simulink model "hybrid_new_eq_circuit_pascal5_single_shot_stack"  (R2019a)
settings: Solver=FixedStepAuto  StartTime=0.0  StopTime=sim_time  FixedStep=resolution  MinStep=0.001  RelTol=1e-4  EnableMultiTasking=on
values from neighbouring files (symbols this model uses):
  amps_in = double(amps_in)    [Sc.m]    (also in sc_model_single_shot_stack.m; test.m = 0; workspace_nedc_basic_sc.mat = 0; workspace_test_model.mat = 0)
  batt_c = [0.25 0.25 0.25 0.25 0.25 0.25 0.25]    [workspace_test_model.mat]
  batt_r = [1 1 1 1 1 1 1 1]    [workspace_test_model.mat]
  resolution = double(resolution)    [Sc.m]    (also in sc_model_single_shot.m = 0.1; sc_model_single_shot_stack.m = 0.1; workspace_test_model.mat = 10)
  tStep = resolution    (= 0.1)    [Sc.m]    (also in testHyb.m = 10; workspace_test_model.mat = 10)
undefined symbols (not defined in the file or in its folder): cCap, cR
libraries: powerlib x525, simulink x9
(part 1 of 8)
settings Model: Creator=ttsh  LastModifiedBy=ttsh
settings SolverCC: ZeroCrossAlgorithm=Adaptive  AlgebraicLoopSolver=LineSearch  SolverResetMethod=Robust
settings DataIOCC: LimitDataPoints=on  SaveFormat=Array  ReturnWorkspaceOutputs=off
settings OptimizationCC: LifeSpan=inf
settings DebuggingCC: SolverPrmCheckMsg=warning  UnconnectedInputMsg=none  UnconnectedOutputMsg=none  UnconnectedLineMsg=none  AllowSymbolicDim=off  SFUnexpectedBacktrackingDiag=warning  SFNoUnconditionalDefaultTransitionDiag=warning  SFExecutionAtInitializationDiag=none  ArithmeticOperatorsInVariantConditions=warning
settings HardwareCC: ProdBitPerPointer=32  ProdBitPerSizeT=32  ProdBitPerPtrDiffT=32  ProdLargestAtomicFloat=None  ProdIntDivRoundTo=Undefined  ProdEndianess=Unspecified  ProdWordSize=32  ProdHWDeviceType=32-bit Generic
settings ModelReferenceCC: PropagateSignalLabelsOutOfModel=off
settings SFSimCC: SimUseLocalCustomCode=off
settings RTWCC: RTWUseLocalCustomCode=off
settings CodeAppCC: StateflowObjectComments=on
settings GRTTargetCC: TargetLangStandard=C89/C90 (ANSI)  GeneratePreprocessorConditionals=Disable all
settings ConfigComp: CovMetricSettings=dw  CovHtmlReporting=on  CovSaveCumulativeToWorkspaceVar=on  CovSaveSingleToWorkspaceVar=on  CovExternalEMLEnable=off  CovSFcnEnable=off
settings SimscapeCC: SimscapeNormalizeSystem=off

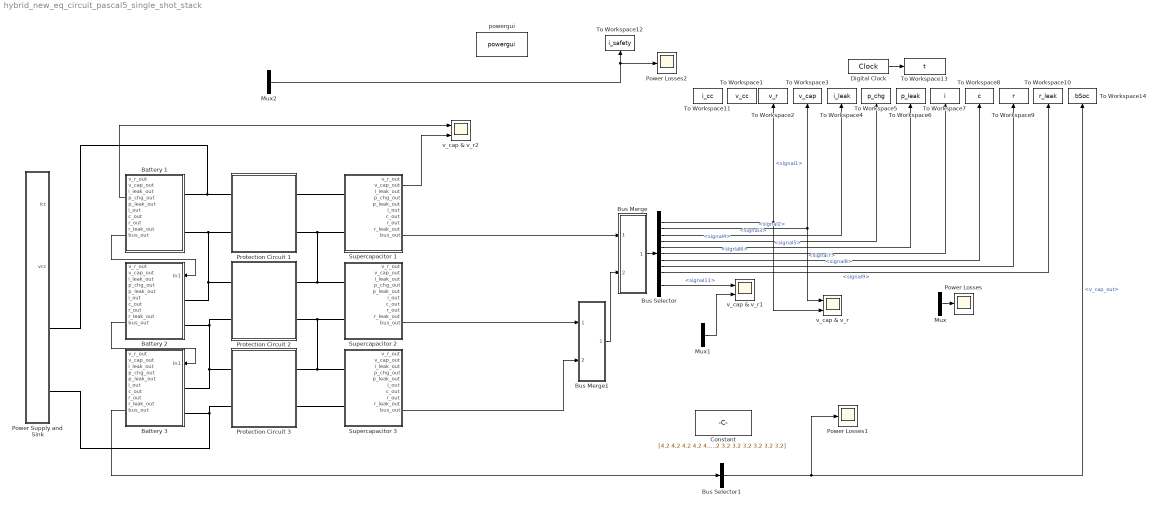
== system hybrid_new_eq_circuit_pascal5_single_shot_stack ==
  Battery 1 : Subsystem  mask{r=batt_r, c=batt_c, v_init=bv_init(end, :, 1), r_leak=inf}
      mask prompts: r "R /ohm (inf for disabled)"; c "Capacitance /F"; v_init "Initial capacitor voltage"; r_leak "R Leak (inf for disabled)"
  Battery 2 : Subsystem  mask{r=batt_r, c=batt_c, v_init=bv_init(end, :, 2), r_leak=inf}
      mask prompts: r "R /ohm (inf for disabled)"; c "Capacitance /F"; v_init "Initial capacitor voltage"; r_leak "R Leak (inf for disabled)"
  Battery 3 : Subsystem  mask{r=batt_r, c=batt_c, v_init=bv_init(end, :, 3), r_leak=inf}
      mask prompts: r "R /ohm (inf for disabled)"; c "Capacitance /F"; v_init "Initial capacitor voltage"; r_leak "R Leak (inf for disabled)"
  Bus Selector : BusSelector  OutputSignals=signal1,signal2,signal3,signal4,signal5,signal6,signal7,signal8,signal9,signal10,signal11
  Bus Selector1 : BusSelector  OutputSignals=v_cap_out
  Bus Merge : Subsystem
  Bus Merge1 : Subsystem
  Constant : Constant  Value=[4.2 4.2 4.2 4.2 4.2 4.2 4.2 4.2 4.2 4.2 4.2 4.2 4.2 4.2 3.2 3.2 3.2 3.2 3.2 3.2 3.2]
  Digital Clock : DigitalClock  SampleTime=resolution
  Mux : Mux  Inputs=2
  Mux1 : Mux  Inputs=2
  Mux2 : Mux  Inputs=3
  Power Losses : Scope
  Power Losses1 : Scope
  Power Losses2 : Scope
  Power Supply and Sink : Subsystem  mask{v_ovp=24}
      mask prompts: v_ovp "V OVP"
  Protection Circuit 1 : Subsystem  mask{r=10, d=0.01, v_cut=8.1, v_min=0, k=off}
      mask prompts: r "Series resistance"; d "Rate limit"; v_cut "v cutoff"; v_min "v min"; k "Enable"
  Protection Circuit 2 : Subsystem  mask{r=10, d=0.01, v_cut=8.1, v_min=0, k=off}
      mask prompts: r "Series resistance"; d "Rate limit"; v_cut "v cutoff"; v_min "v min"; k "Enable"
  Protection Circuit 3 : Subsystem  mask{r=10, d=0.01, v_cut=8.1, v_min=0, k=off}
      mask prompts: r "Series resistance"; d "Rate limit"; v_cut "v cutoff"; v_min "v min"; k "Enable"
  Supercapacitor 1 : Subsystem  mask{r_leak=inf, c=cCap, r=cR, ord=5, v_init1=v_init(end, 1, 1), v_init2=v_init(end, 2, 1), v_init3=v_init(end, 3, 1), v_init4=v_init(end, 4, 1), v_init5=v_init(end, 5, 1)}
      mask prompts: r_leak "R Leak /ohm (inf for disabled)"; c "Capacitance /F"; r "Resistance"; ord "Elements (pascal order)"; v_init1 "Initial capacitor voltage"; v_init2 "Initial capacitor voltage"; v_init3 "Initial capacitor voltage"; v_init4 "Initial capacitor voltage"; v_init5 "Initial capacitor voltage"
  Supercapacitor 2 : Subsystem  mask{r_leak=inf, c=cCap, r=cR, ord=5, v_init1=v_init(end, 1, 2), v_init2=v_init(end, 2, 2), v_init3=v_init(end, 3, 2), v_init4=v_init(end, 4, 2), v_init5=v_init(end, 5, 2)}
      mask prompts: r_leak "R Leak /ohm (inf for disabled)"; c "Capacitance /F"; r "Resistance"; ord "Elements (pascal order)"; v_init1 "Initial capacitor voltage"; v_init2 "Initial capacitor voltage"; v_init3 "Initial capacitor voltage"; v_init4 "Initial capacitor voltage"; v_init5 "Initial capacitor voltage"
  Supercapacitor 3 : Subsystem  mask{r_leak=inf, c=cCap, r=cR, ord=5, v_init1=v_init(end, 1, 3), v_init2=v_init(end, 2, 3), v_init3=v_init(end, 3, 3), v_init4=v_init(end, 4, 3), v_init5=v_init(end, 5, 3)}
      mask prompts: r_leak "R Leak /ohm (inf for disabled)"; c "Capacitance /F"; r "Resistance"; ord "Elements (pascal order)"; v_init1 "Initial capacitor voltage"; v_init2 "Initial capacitor voltage"; v_init3 "Initial capacitor voltage"; v_init4 "Initial capacitor voltage"; v_init5 "Initial capacitor voltage"
  To Workspace1 : ToWorkspace  VariableName=v_cc  SampleTime=-1
      settings: Save2DSignal=2-D array (concatenate along first dimension)
  To Workspace10 : ToWorkspace  VariableName=r_leak  SampleTime=-1
  To Workspace11 : ToWorkspace  VariableName=i_cc  SampleTime=-1
      settings: Save2DSignal=2-D array (concatenate along first dimension)
  To Workspace12 : ToWorkspace  VariableName=i_safety  SampleTime=-1
      settings: Save2DSignal=2-D array (concatenate along first dimension)
  To Workspace13 : ToWorkspace  VariableName=t  SampleTime=-1
      settings: Save2DSignal=2-D array (concatenate along first dimension)
  To Workspace14 : ToWorkspace  VariableName=bSoc  SampleTime=-1
  To Workspace2 : ToWorkspace  VariableName=v_r  SampleTime=-1
  To Workspace3 : ToWorkspace  VariableName=v_cap  SampleTime=-1
  To Workspace4 : ToWorkspace  VariableName=i_leak  SampleTime=-1
  To Workspace5 : ToWorkspace  VariableName=p_chg  SampleTime=-1
  To Workspace6 : ToWorkspace  VariableName=p_leak  SampleTime=-1
  To Workspace7 : ToWorkspace  VariableName=i  SampleTime=-1
  To Workspace8 : ToWorkspace  VariableName=c  SampleTime=-1
  To Workspace9 : ToWorkspace  VariableName=r  SampleTime=-1
  powergui : powerlib/powergui  Priority=1  SimulationMode=Discrete  SampleTime=tStep  frequency=60  Iterations=50  frequencyindice=0  Pbase=100e6  ErrMax=1e-4  UnitsV=V  UnitsW=W  buscounter=0  FunctionMessages=on  echomessages=off  EnableUseOfTLC=off  CurrentSourceSwitches=on  DisableSnubberDevices=on  DisableRonSwitches=on  DisableVfSwitches=on  DisplayEquations=off  AutomaticDiscreteSolvers=off  SolverType=Tustin  Interpol=off  ExternalGateDelay=off  methode=off  Ts=0  x0status=blocks  SPID=off  SwTol=0  HookPort=off  NonlinearTolerance=0  nMaxIteration=15  ContinueOnMaxIteration=off  RestoreLinks=warning  ResistiveCurrentMeasurement=off  Frange=[0:2:500]  Ylog=off  Xlog=on  ShowGrid=off  save=off  variable=ZData  structure=0  ZoomFFT=off  StartTime=0.0  cycles=1  DisplayStyle=1  fundamental=60  FreqAxis=off  MaxFrequency=1000  frequencyindicesteady=1  RmsSteady=1  display=off
      settings: SourceProductName=Simscape Electrical
  v_cap & v_r : Scope  NumInputPorts=2
  v_cap & v_r1 : Scope  NumInputPorts=2
  v_cap & v_r2 : Scope  NumInputPorts=2
  wires:
  Mux/1 -> Power Losses/1
  Supercapacitor 1/10(bus_out) -> Bus Merge/1(bus_1_in)
  Bus Merge/1(bus_out) -> Bus Selector/1
  Bus Selector/1 -> v_cap & v_r/2, To Workspace2/1  "<signal1>"
  Bus Selector/2 -> v_cap & v_r/1, To Workspace3/1  "<signal2>"
  Bus Selector/3 -> To Workspace4/1  "<signal3>"
  Bus Selector/4 -> To Workspace5/1  "<signal4>"
  Bus Selector/5 -> To Workspace6/1  "<signal5>"
  Bus Selector/6 -> To Workspace7/1  "<signal6>"
  Bus Selector/7 -> To Workspace8/1  "<signal7>"
  Bus Selector/8 -> To Workspace9/1  "<signal8>"
  Bus Selector/9 -> To Workspace10/1  "<signal9>"
  Bus Selector/11 -> v_cap & v_r1/1  "<signal11>"
  Supercapacitor 2/10(bus_out) -> Bus Merge1/1(bus_1_in)
  Supercapacitor 3/10(bus_out) -> Bus Merge1/2(bus_2_in)
  Bus Merge1/1(bus_out) -> Bus Merge/2(bus_2_in)
  Mux1/1 -> v_cap & v_r1/2
  Mux2/1 -> Power Losses2/1, To Workspace12/1
  Digital Clock/1 -> To Workspace13/1
  Supercapacitor 1/2(v_cap_out) -> v_cap & v_r2/2
  Battery 1/4(p_chg_out) -> v_cap & v_r2/1
  Battery 1/10(bus_out) -> Battery 2/1(In1)
  Battery 2/10(bus_out) -> Battery 3/1(In1)
  Battery 3/10(bus_out) -> Bus Selector1/1
  Bus Selector1/1 -> To Workspace14/1, Power Losses1/1  "<v_cap_out>"
  connections:
  Power Supply and Sink/RConn1 -- Battery 1/LConn1 -- Protection Circuit 1/LConn1
  Protection Circuit 2/LConn1 -- Battery 1/LConn2 -- Protection Circuit 1/LConn2 -- Battery 2/LConn1
  Protection Circuit 1/RConn1 -- Supercapacitor 1/LConn1
  Protection Circuit 2/RConn1 -- Supercapacitor 2/LConn1 -- Supercapacitor 1/LConn2 -- Protection Circuit 1/RConn2
  Protection Circuit 2/LConn2 -- Battery 2/LConn2 -- Battery 3/LConn1 -- Protection Circuit 3/LConn1
  Power Supply and Sink/RConn2 -- Battery 3/LConn2 -- Protection Circuit 3/LConn2
  Protection Circuit 2/RConn2 -- Supercapacitor 2/LConn2 -- Supercapacitor 3/LConn1 -- Protection Circuit 3/RConn1
  Supercapacitor 3/LConn2 -- Protection Circuit 3/RConn2

== system hybrid_new_eq_circuit_pascal5_single_shot_stack/Battery 1 ==
  note: 1x 550R
  Bus Creator : BusCreator  Inputs=11
  Constant : Constant
  Series RLC Branch1 : powerlib/Elements/Series RLC Branch  LConnTagsString=__new0  RConnTagsString=__new0  BranchType=R  Resistance=r(8)  Inductance=1e-3  SetiL0=off  InitialCurrent=0  Capacitance=1e-6  Setx0=off  InitialVoltage=0  Measurements=None
      settings: SourceProductName=Simscape Electrical
  Series RLC Branch2 : powerlib/Elements/Series RLC Branch  LConnTagsString=__new0  RConnTagsString=__new0  BranchType=R  Resistance=r(1)  Inductance=1e-3  SetiL0=off  InitialCurrent=0  Capacitance=1e-6  Setx0=off  InitialVoltage=0  Measurements=None
      settings: SourceProductName=Simscape Electrical
  Series RLC Branch3 : powerlib/Elements/Series RLC Branch  LConnTagsString=__new0  RConnTagsString=__new0  BranchType=R  Resistance=r(2)  Inductance=1e-3  SetiL0=off  InitialCurrent=0  Capacitance=1e-6  Setx0=off  InitialVoltage=0  Measurements=None
      settings: SourceProductName=Simscape Electrical
  Series RLC Branch4 : powerlib/Elements/Series RLC Branch  LConnTagsString=__new0  RConnTagsString=__new0  BranchType=R  Resistance=r(3)  Inductance=1e-3  SetiL0=off  InitialCurrent=0  Capacitance=1e-6  Setx0=off  InitialVoltage=0  Measurements=None
      settings: SourceProductName=Simscape Electrical
  Subsystem : Subsystem  mask{c=c, r=r, r_leak=r_leak, v_init=v_init}
      mask prompts: c "Capacitance /F"; r "Series resistance /ohm"; r_leak "Leak resistance /ohm (inf for disabled)"; v_init "Initial capacitor voltage"
  Subsystem3 : Subsystem  mask{c=c(2), r_esr=0.001, r_leak=r_leak, v_init=v_init(2)}
      mask prompts: c "Capacitance /F"; r_esr "Series resistance /ohm"; r_leak "Leakage resistance /ohm (inf for disabled)"; v_init "Initial capacitor voltage"
  Subsystem4 : Subsystem  mask{c=c(3), r_esr=0.001, r_leak=r_leak, v_init=v_init(3)}
      mask prompts: c "Capacitance /F"; r_esr "Series resistance /ohm"; r_leak "Leakage resistance /ohm (inf for disabled)"; v_init "Initial capacitor voltage"
  Subsystem8 : Subsystem  mask{c=c(1), r_esr=0.001, r_leak=r_leak, v_init=v_init(1)}
      mask prompts: c "Capacitance /F"; r_esr "Series resistance /ohm"; r_leak "Leakage resistance /ohm (inf for disabled)"; v_init "Initial capacitor voltage"
  v_cap : Scope
  v_cap_single : powerlib/Measurements/Voltage Measurement  PhasorSimulation=off  OutputType=Complex  PSBequivalent=0
      settings: SourceProductName=Simscape Electrical
  VCC_in : PMIOPort  Side=Left
  VSS_in : PMIOPort  Port=2  Side=Left
  VCC_out : PMIOPort  Port=3  Side=Right
  VSS_out : PMIOPort  Port=4  Side=Right
  v_r_out : Outport
  v_cap_out : Outport  Port=2
  i_leak_out : Outport  Port=3
  p_chg_out : Outport  Port=4
  p_leak_out : Outport  Port=5
  i_out : Outport  Port=6
  c_out : Outport  Port=7
  r_out : Outport  Port=8
  r_leak_out : Outport  Port=9
  bus_out : Outport  Port=10
  wires:
  Subsystem/10(Out10) -> Bus Creator/10
  v_cap_single/1 -> Bus Creator/11
  Subsystem/1(Out1) -> v_r_out/1, Bus Creator/1
  Subsystem/9(Out9) -> r_leak_out/1, Bus Creator/9
  Subsystem/2(Out2) -> v_cap_out/1, v_cap/1, Bus Creator/2  "v_cap_out"
  Subsystem/8(Out8) -> r_out/1, Bus Creator/8
  Subsystem/3(Out3) -> i_leak_out/1, Bus Creator/3
  Subsystem/7(Out7) -> c_out/1, Bus Creator/7
  Subsystem/4(Out4) -> p_chg_out/1, Bus Creator/4
  Subsystem/6(Out6) -> i_out/1, Bus Creator/6
  Subsystem/5(Out5) -> p_leak_out/1, Bus Creator/5
  Subsystem8/1(v_r_out) -> Subsystem3/1(v_r_in)
  Subsystem8/3(i_leak_out) -> Subsystem3/3(i_leak_in)
  Subsystem8/4(p_chg_out) -> Subsystem3/4(p_chg_in)
  Subsystem8/5(p_leak_out) -> Subsystem3/5(p_leak_in)
  Subsystem8/6(i_out) -> Subsystem3/6(i_in)
  Subsystem8/7(c_out) -> Subsystem3/7(c_in)
  Subsystem8/8(r_out) -> Subsystem3/8(r_in)
  Subsystem8/9(r_leak_out) -> Subsystem3/9(r_leak_in)
  Subsystem8/10(l_out) -> Subsystem3/10(l_in)
  Subsystem3/1(v_r_out) -> Subsystem4/1(v_r_in)
  Subsystem3/3(i_leak_out) -> Subsystem4/3(i_leak_in)
  Subsystem3/4(p_chg_out) -> Subsystem4/4(p_chg_in)
  Subsystem3/5(p_leak_out) -> Subsystem4/5(p_leak_in)
  Subsystem3/6(i_out) -> Subsystem4/6(i_in)
  Subsystem3/7(c_out) -> Subsystem4/7(c_in)
  Subsystem3/8(r_out) -> Subsystem4/8(r_in)
  Subsystem3/9(r_leak_out) -> Subsystem4/9(r_leak_in)
  Subsystem3/10(l_out) -> Subsystem4/10(l_in)
  Subsystem4/1(v_r_out) -> Subsystem/1(In1)
  Subsystem4/3(i_leak_out) -> Subsystem/3(In3)
  Subsystem4/4(p_chg_out) -> Subsystem/4(In4)
  Subsystem4/5(p_leak_out) -> Subsystem/5(In5)
  Subsystem4/6(i_out) -> Subsystem/6(In6)
  Subsystem4/7(c_out) -> Subsystem/7(In7)
  Subsystem4/8(r_out) -> Subsystem/8(In8)
  Subsystem4/9(r_leak_out) -> Subsystem/9(In9)
  Subsystem4/10(l_out) -> Subsystem/10(In10)
  Bus Creator/1 -> bus_out/1
  Subsystem3/2(v_cap_out) -> Subsystem4/2(v_cap_in)  "v_cap_out"
  Subsystem4/2(v_cap_out) -> Subsystem/2(In2)  "v_cap_out"
  Subsystem8/2(v_cap_out) -> Subsystem3/2(v_cap_in)  "v_cap_out"
  connections:
  VSS_out/RConn1 -- VSS_in/RConn1 -- Subsystem/RConn2 -- v_cap_single/LConn2
  Subsystem8/LConn1 -- Series RLC Branch2/RConn1 -- Series RLC Branch1/LConn1
  VCC_out/RConn1 -- v_cap_single/LConn1 -- VCC_in/RConn1
  Series RLC Branch3/RConn1 -- Subsystem3/LConn1 -- Subsystem8/RConn2 -- Series RLC Branch2/LConn1
  Series RLC Branch3/LConn1 -- Subsystem4/LConn1 -- Subsystem3/RConn2 -- Series RLC Branch4/RConn1
  Subsystem4/RConn2 -- Subsystem/LConn1 -- Series RLC Branch4/LConn1

== system hybrid_new_eq_circuit_pascal5_single_shot_stack/Battery 2 ==
  note: 1x 550R
  In1 : Inport
  Bus Creator : BusCreator  Inputs=11
  Bus Merge2 : Subsystem
  Series RLC Branch1 : powerlib/Elements/Series RLC Branch  LConnTagsString=__new0  RConnTagsString=__new0  BranchType=R  Resistance=r(8)  Inductance=1e-3  SetiL0=off  InitialCurrent=0  Capacitance=1e-6  Setx0=off  InitialVoltage=0  Measurements=None
      settings: SourceProductName=Simscape Electrical
  Series RLC Branch2 : powerlib/Elements/Series RLC Branch  LConnTagsString=__new0  RConnTagsString=__new0  BranchType=R  Resistance=r(1)  Inductance=1e-3  SetiL0=off  InitialCurrent=0  Capacitance=1e-6  Setx0=off  InitialVoltage=0  Measurements=None
      settings: SourceProductName=Simscape Electrical
  Series RLC Branch3 : powerlib/Elements/Series RLC Branch  LConnTagsString=__new0  RConnTagsString=__new0  BranchType=R  Resistance=r(2)  Inductance=1e-3  SetiL0=off  InitialCurrent=0  Capacitance=1e-6  Setx0=off  InitialVoltage=0  Measurements=None
      settings: SourceProductName=Simscape Electrical
  Series RLC Branch4 : powerlib/Elements/Series RLC Branch  LConnTagsString=__new0  RConnTagsString=__new0  BranchType=R  Resistance=r(3)  Inductance=1e-3  SetiL0=off  InitialCurrent=0  Capacitance=1e-6  Setx0=off  InitialVoltage=0  Measurements=None
      settings: SourceProductName=Simscape Electrical
  Subsystem : Subsystem  mask{c=c, r=r, r_leak=r_leak, v_init=v_init}
      mask prompts: c "Capacitance /F"; r "Series resistance /ohm"; r_leak "Leak resistance /ohm (inf for disabled)"; v_init "Initial capacitor voltage"
  Subsystem3 : Subsystem  mask{c=c(2), r_esr=0.001, r_leak=r_leak, v_init=v_init(2)}
      mask prompts: c "Capacitance /F"; r_esr "Series resistance /ohm"; r_leak "Leakage resistance /ohm (inf for disabled)"; v_init "Initial capacitor voltage"
  Subsystem4 : Subsystem  mask{c=c(3), r_esr=0.001, r_leak=r_leak, v_init=v_init(3)}
      mask prompts: c "Capacitance /F"; r_esr "Series resistance /ohm"; r_leak "Leakage resistance /ohm (inf for disabled)"; v_init "Initial capacitor voltage"
  Subsystem8 : Subsystem  mask{c=c(1), r_esr=0.001, r_leak=r_leak, v_init=v_init(1)}
      mask prompts: c "Capacitance /F"; r_esr "Series resistance /ohm"; r_leak "Leakage resistance /ohm (inf for disabled)"; v_init "Initial capacitor voltage"
  v_cap_single : powerlib/Measurements/Voltage Measurement  PhasorSimulation=off  OutputType=Complex  PSBequivalent=0
      settings: SourceProductName=Simscape Electrical
  VCC_in : PMIOPort  Side=Left
  VSS_in : PMIOPort  Port=2  Side=Left
  VCC_out : PMIOPort  Port=3  Side=Right
  VSS_out : PMIOPort  Port=4  Side=Right
  v_r_out : Outport
  v_cap_out : Outport  Port=2
  i_leak_out : Outport  Port=3
  p_chg_out : Outport  Port=4
  p_leak_out : Outport  Port=5
  i_out : Outport  Port=6
  c_out : Outport  Port=7
  r_out : Outport  Port=8
  r_leak_out : Outport  Port=9
  bus_out : Outport  Port=10
  wires:
  Bus Merge2/1(bus_out) -> bus_out/1
  In1/1 -> Bus Merge2/1(bus_1_in)
  Subsystem4/10(l_out) -> Subsystem/10(In10)
  Subsystem4/9(r_leak_out) -> Subsystem/9(In9)
  Subsystem4/8(r_out) -> Subsystem/8(In8)
  Subsystem4/7(c_out) -> Subsystem/7(In7)
  Subsystem4/6(i_out) -> Subsystem/6(In6)
  Subsystem4/5(p_leak_out) -> Subsystem/5(In5)
  Subsystem4/4(p_chg_out) -> Subsystem/4(In4)
  Subsystem4/3(i_leak_out) -> Subsystem/3(In3)
  Subsystem4/2(v_cap_out) -> Subsystem/2(In2)
  Subsystem4/1(v_r_out) -> Subsystem/1(In1)
  Subsystem3/10(l_out) -> Subsystem4/10(l_in)
  Subsystem3/9(r_leak_out) -> Subsystem4/9(r_leak_in)
  Subsystem3/8(r_out) -> Subsystem4/8(r_in)
  Subsystem3/7(c_out) -> Subsystem4/7(c_in)
  Subsystem3/6(i_out) -> Subsystem4/6(i_in)
  Subsystem3/5(p_leak_out) -> Subsystem4/5(p_leak_in)
  Subsystem3/4(p_chg_out) -> Subsystem4/4(p_chg_in)
  Subsystem3/3(i_leak_out) -> Subsystem4/3(i_leak_in)
  Subsystem3/2(v_cap_out) -> Subsystem4/2(v_cap_in)
  Subsystem3/1(v_r_out) -> Subsystem4/1(v_r_in)
  Subsystem8/10(l_out) -> Subsystem3/10(l_in)
  Subsystem8/9(r_leak_out) -> Subsystem3/9(r_leak_in)
  Subsystem8/8(r_out) -> Subsystem3/8(r_in)
  Subsystem8/7(c_out) -> Subsystem3/7(c_in)
  Subsystem8/6(i_out) -> Subsystem3/6(i_in)
  Subsystem8/5(p_leak_out) -> Subsystem3/5(p_leak_in)
  Subsystem8/4(p_chg_out) -> Subsystem3/4(p_chg_in)
  Subsystem8/3(i_leak_out) -> Subsystem3/3(i_leak_in)
  Subsystem8/2(v_cap_out) -> Subsystem3/2(v_cap_in)
  Subsystem8/1(v_r_out) -> Subsystem3/1(v_r_in)
  Subsystem/5(Out5) -> Bus Creator/5, p_leak_out/1
  Subsystem/6(Out6) -> Bus Creator/6, i_out/1
  Subsystem/4(Out4) -> Bus Creator/4, p_chg_out/1
  Subsystem/7(Out7) -> Bus Creator/7, c_out/1
  Subsystem/3(Out3) -> Bus Creator/3, i_leak_out/1
  Subsystem/8(Out8) -> Bus Creator/8, r_out/1
  Subsystem/2(Out2) -> Bus Creator/2, v_cap_out/1  "v_cap_out"
  Subsystem/9(Out9) -> Bus Creator/9, r_leak_out/1
  Subsystem/1(Out1) -> Bus Creator/1, v_r_out/1
  v_cap_single/1 -> Bus Creator/11
  Subsystem/10(Out10) -> Bus Creator/10
  Bus Creator/1 -> Bus Merge2/2(bus_2_in)
  connections:
  VCC_out/RConn1 -- VCC_in/RConn1 -- Series RLC Branch1/RConn1 -- v_cap_single/LConn1
  Subsystem8/LConn1 -- Series RLC Branch1/LConn1 -- Series RLC Branch2/RConn1
  v_cap_single/LConn2 -- VSS_in/RConn1 -- Subsystem/RConn2 -- VSS_out/RConn1
  Series RLC Branch3/RConn1 -- Subsystem8/RConn2 -- Subsystem3/LConn1 -- Series RLC Branch2/LConn1
  Series RLC Branch3/LConn1 -- Subsystem4/LConn1 -- Subsystem3/RConn2 -- Series RLC Branch4/RConn1
  Subsystem4/RConn2 -- Series RLC Branch4/LConn1 -- Subsystem/LConn1

== system hybrid_new_eq_circuit_pascal5_single_shot_stack/Battery 3 ==
  note: 1x 550R
  In1 : Inport
  Bus Creator : BusCreator  Inputs=11
  Bus Merge2 : Subsystem
  Series RLC Branch1 : powerlib/Elements/Series RLC Branch  LConnTagsString=__new0  RConnTagsString=__new0  BranchType=R  Resistance=r(8)  Inductance=1e-3  SetiL0=off  InitialCurrent=0  Capacitance=1e-6  Setx0=off  InitialVoltage=0  Measurements=None
      settings: SourceProductName=Simscape Electrical
  Series RLC Branch2 : powerlib/Elements/Series RLC Branch  LConnTagsString=__new0  RConnTagsString=__new0  BranchType=R  Resistance=r(1)  Inductance=1e-3  SetiL0=off  InitialCurrent=0  Capacitance=1e-6  Setx0=off  InitialVoltage=0  Measurements=None
      settings: SourceProductName=Simscape Electrical
  Series RLC Branch3 : powerlib/Elements/Series RLC Branch  LConnTagsString=__new0  RConnTagsString=__new0  BranchType=R  Resistance=r(2)  Inductance=1e-3  SetiL0=off  InitialCurrent=0  Capacitance=1e-6  Setx0=off  InitialVoltage=0  Measurements=None
      settings: SourceProductName=Simscape Electrical
  Series RLC Branch4 : powerlib/Elements/Series RLC Branch  LConnTagsString=__new0  RConnTagsString=__new0  BranchType=R  Resistance=r(3)  Inductance=1e-3  SetiL0=off  InitialCurrent=0  Capacitance=1e-6  Setx0=off  InitialVoltage=0  Measurements=None
      settings: SourceProductName=Simscape Electrical
  Subsystem : Subsystem  mask{c=c, r=r, r_leak=r_leak, v_init=v_init}
      mask prompts: c "Capacitance /F"; r "Series resistance /ohm"; r_leak "Leak resistance /ohm (inf for disabled)"; v_init "Initial capacitor voltage"
  Subsystem3 : Subsystem  mask{c=c(2), r_esr=0.001, r_leak=r_leak, v_init=v_init(2)}
      mask prompts: c "Capacitance /F"; r_esr "Series resistance /ohm"; r_leak "Leakage resistance /ohm (inf for disabled)"; v_init "Initial capacitor voltage"
  Subsystem4 : Subsystem  mask{c=c(3), r_esr=0.001, r_leak=r_leak, v_init=v_init(3)}
      mask prompts: c "Capacitance /F"; r_esr "Series resistance /ohm"; r_leak "Leakage resistance /ohm (inf for disabled)"; v_init "Initial capacitor voltage"
  Subsystem8 : Subsystem  mask{c=c(1), r_esr=0.001, r_leak=r_leak, v_init=v_init(1)}
      mask prompts: c "Capacitance /F"; r_esr "Series resistance /ohm"; r_leak "Leakage resistance /ohm (inf for disabled)"; v_init "Initial capacitor voltage"
  v_cap_single : powerlib/Measurements/Voltage Measurement  PhasorSimulation=off  OutputType=Complex  PSBequivalent=0
      settings: SourceProductName=Simscape Electrical
  VCC_in : PMIOPort  Side=Left
  VSS_in : PMIOPort  Port=2  Side=Left
  VCC_out : PMIOPort  Port=3  Side=Right
  VSS_out : PMIOPort  Port=4  Side=Right
  v_r_out : Outport
  v_cap_out : Outport  Port=2
  i_leak_out : Outport  Port=3
  p_chg_out : Outport  Port=4
  p_leak_out : Outport  Port=5
  i_out : Outport  Port=6
  c_out : Outport  Port=7
  r_out : Outport  Port=8
  r_leak_out : Outport  Port=9
  bus_out : Outport  Port=10
  wires:
  Bus Merge2/1(bus_out) -> bus_out/1
  In1/1 -> Bus Merge2/1(bus_1_in)
  Subsystem4/10(l_out) -> Subsystem/10(In10)
  Subsystem4/9(r_leak_out) -> Subsystem/9(In9)
  Subsystem4/8(r_out) -> Subsystem/8(In8)
  Subsystem4/7(c_out) -> Subsystem/7(In7)
  Subsystem4/6(i_out) -> Subsystem/6(In6)
  Subsystem4/5(p_leak_out) -> Subsystem/5(In5)
  Subsystem4/4(p_chg_out) -> Subsystem/4(In4)
  Subsystem4/3(i_leak_out) -> Subsystem/3(In3)
  Subsystem4/2(v_cap_out) -> Subsystem/2(In2)
  Subsystem4/1(v_r_out) -> Subsystem/1(In1)
  Subsystem3/10(l_out) -> Subsystem4/10(l_in)
  Subsystem3/9(r_leak_out) -> Subsystem4/9(r_leak_in)
  Subsystem3/8(r_out) -> Subsystem4/8(r_in)
  Subsystem3/7(c_out) -> Subsystem4/7(c_in)
  Subsystem3/6(i_out) -> Subsystem4/6(i_in)
  Subsystem3/5(p_leak_out) -> Subsystem4/5(p_leak_in)
  Subsystem3/4(p_chg_out) -> Subsystem4/4(p_chg_in)
  Subsystem3/3(i_leak_out) -> Subsystem4/3(i_leak_in)
  Subsystem3/2(v_cap_out) -> Subsystem4/2(v_cap_in)
  Subsystem3/1(v_r_out) -> Subsystem4/1(v_r_in)
  Subsystem8/10(l_out) -> Subsystem3/10(l_in)
  Subsystem8/9(r_leak_out) -> Subsystem3/9(r_leak_in)
  Subsystem8/8(r_out) -> Subsystem3/8(r_in)
  Subsystem8/7(c_out) -> Subsystem3/7(c_in)
  Subsystem8/6(i_out) -> Subsystem3/6(i_in)
  Subsystem8/5(p_leak_out) -> Subsystem3/5(p_leak_in)
  Subsystem8/4(p_chg_out) -> Subsystem3/4(p_chg_in)
  Subsystem8/3(i_leak_out) -> Subsystem3/3(i_leak_in)
  Subsystem8/2(v_cap_out) -> Subsystem3/2(v_cap_in)
  Subsystem8/1(v_r_out) -> Subsystem3/1(v_r_in)
  Subsystem/5(Out5) -> Bus Creator/5, p_leak_out/1
  Subsystem/6(Out6) -> Bus Creator/6, i_out/1
  Subsystem/4(Out4) -> Bus Creator/4, p_chg_out/1
  Subsystem/7(Out7) -> Bus Creator/7, c_out/1
  Subsystem/3(Out3) -> Bus Creator/3, i_leak_out/1
  Subsystem/8(Out8) -> Bus Creator/8, r_out/1
  Subsystem/2(Out2) -> Bus Creator/2, v_cap_out/1  "v_cap_out"
  Subsystem/9(Out9) -> Bus Creator/9, r_leak_out/1
  Subsystem/1(Out1) -> Bus Creator/1, v_r_out/1
  v_cap_single/1 -> Bus Creator/11
  Subsystem/10(Out10) -> Bus Creator/10
  Bus Creator/1 -> Bus Merge2/2(bus_2_in)
  connections:
  Subsystem8/LConn1 -- Series RLC Branch2/RConn1 -- Series RLC Branch1/LConn1
  v_cap_single/LConn2 -- VSS_in/RConn1 -- Subsystem/RConn2 -- VSS_out/RConn1
  Series RLC Branch1/RConn1 -- v_cap_single/LConn1 -- VCC_out/RConn1 -- VCC_in/RConn1
  Series RLC Branch3/RConn1 -- Subsystem3/LConn1 -- Subsystem8/RConn2 -- Series RLC Branch2/LConn1
  Series RLC Branch3/LConn1 -- Subsystem4/LConn1 -- Subsystem3/RConn2 -- Series RLC Branch4/RConn1
  Subsystem4/RConn2 -- Series RLC Branch4/LConn1 -- Subsystem/LConn1

== system hybrid_new_eq_circuit_pascal5_single_shot_stack/Bus Merge ==
  bus_1_in : Inport
  bus_2_in : Inport  Port=2
  Bus Creator : BusCreator  Inputs=11
  Bus Selector : BusSelector  OutputSignals=signal1,signal2,signal3,signal4,signal5,signal6,signal7,signal8,signal9,signal10,signal11
  Bus Selector1 : BusSelector  OutputSignals=signal1,signal2,signal3,signal4,signal5,signal6,signal7,signal8,signal9,signal10,signal11
  Mux{1..11} (11 alike) : Mux  Inputs=2
  bus_out : Outport
  wires:
  bus_1_in/1 -> Bus Selector/1
  bus_2_in/1 -> Bus Selector1/1
  Bus Creator/1 -> bus_out/1
  Bus Selector/1 -> Mux1/1  "<signal1>"
  Bus Selector1/2 -> Mux2/2  "<signal2>"
  Bus Selector/3 -> Mux3/1  "<signal3>"
  Bus Selector1/4 -> Mux4/2  "<signal4>"
  Bus Selector/5 -> Mux5/1  "<signal5>"
  Bus Selector1/6 -> Mux6/1  "<signal6>"
  Bus Selector/7 -> Mux7/1  "<signal7>"
  Bus Selector1/8 -> Mux8/1  "<signal8>"
  Bus Selector1/10 -> Mux10/1  "<signal10>"
  Bus Selector/11 -> Mux11/1  "<signal11>"
  Bus Selector/9 -> Mux9/1  "<signal9>"
  Bus Selector/2 -> Mux2/1  "<signal2>"
  Bus Selector/4 -> Mux4/1  "<signal4>"
  Bus Selector/6 -> Mux6/2  "<signal6>"
  Bus Selector/8 -> Mux8/2  "<signal8>"
  Bus Selector/10 -> Mux10/2  "<signal10>"
  Bus Selector1/1 -> Mux1/2  "<signal1>"
  Bus Selector1/3 -> Mux3/2  "<signal3>"
  Bus Selector1/5 -> Mux5/2  "<signal5>"
  Bus Selector1/7 -> Mux7/2  "<signal7>"
  Bus Selector1/9 -> Mux9/2  "<signal9>"
  Bus Selector1/11 -> Mux11/2  "<signal11>"
  Mux1/1 -> Bus Creator/1
  Mux3/1 -> Bus Creator/3
  Mux5/1 -> Bus Creator/5
  Mux7/1 -> Bus Creator/7
  Mux9/1 -> Bus Creator/9
  Mux11/1 -> Bus Creator/11
  Mux2/1 -> Bus Creator/2
  Mux4/1 -> Bus Creator/4
  Mux6/1 -> Bus Creator/6
  Mux8/1 -> Bus Creator/8
  Mux10/1 -> Bus Creator/10

== system hybrid_new_eq_circuit_pascal5_single_shot_stack/Bus Merge1 ==
  bus_1_in : Inport
  bus_2_in : Inport  Port=2
  Bus Creator : BusCreator  Inputs=11
  Bus Selector : BusSelector  OutputSignals=signal1,signal2,signal3,signal4,signal5,signal6,signal7,signal8,signal9,signal10,signal11
  Bus Selector1 : BusSelector  OutputSignals=signal1,signal2,signal3,signal4,signal5,signal6,signal7,signal8,signal9,signal10,signal11
  Mux{1..11} (11 alike) : Mux  Inputs=2
  bus_out : Outport
  wires:
  Mux10/1 -> Bus Creator/10
  Mux8/1 -> Bus Creator/8
  Mux6/1 -> Bus Creator/6
  Mux4/1 -> Bus Creator/4
  Mux2/1 -> Bus Creator/2
  Mux11/1 -> Bus Creator/11
  Mux9/1 -> Bus Creator/9
  Mux7/1 -> Bus Creator/7
  Mux5/1 -> Bus Creator/5
  Mux3/1 -> Bus Creator/3
  Mux1/1 -> Bus Creator/1
  Bus Selector1/11 -> Mux11/2  "<signal11>"
  Bus Selector1/9 -> Mux9/2  "<signal9>"
  Bus Selector1/7 -> Mux7/2  "<signal7>"
  Bus Selector1/5 -> Mux5/2  "<signal5>"
  Bus Selector1/3 -> Mux3/2  "<signal3>"
  Bus Selector1/1 -> Mux1/2  "<signal1>"
  Bus Selector/10 -> Mux10/2  "<signal10>"
  Bus Selector/8 -> Mux8/2  "<signal8>"
  Bus Selector/6 -> Mux6/2  "<signal6>"
  Bus Selector/4 -> Mux4/1  "<signal4>"
  Bus Selector/2 -> Mux2/1  "<signal2>"
  Bus Selector/9 -> Mux9/1  "<signal9>"
  Bus Selector/11 -> Mux11/1  "<signal11>"
  Bus Selector1/10 -> Mux10/1  "<signal10>"
  Bus Selector1/8 -> Mux8/1  "<signal8>"
  Bus Selector/7 -> Mux7/1  "<signal7>"
  Bus Selector1/6 -> Mux6/1  "<signal6>"
  Bus Selector/5 -> Mux5/1  "<signal5>"
  Bus Selector1/4 -> Mux4/2  "<signal4>"
  Bus Selector/3 -> Mux3/1  "<signal3>"
  Bus Selector1/2 -> Mux2/2  "<signal2>"
  Bus Selector/1 -> Mux1/1  "<signal1>"
  Bus Creator/1 -> bus_out/1
  bus_2_in/1 -> Bus Selector1/1
  bus_1_in/1 -> Bus Selector/1

== system hybrid_new_eq_circuit_pascal5_single_shot_stack/Power Supply and Sink ==
  Compare To Zero : simulink/Logic and Bit Operations/Compare To Zero  relop=>  OutDataTypeStr=boolean
  Compare To Zero1 : simulink/Logic and Bit Operations/Compare To Zero  relop=~=  OutDataTypeStr=uint8
  Constant : Constant  Value=3*5
  Constant1 : Constant  Value=amps_in
  Constant2 : Constant  Value=3*5
  Controlled Current Source2 : powerlib/Electrical Sources/Controlled Current Source  Initialize=on  Source_Type=DC  Amplitude=0  Phase=0  Frequency=0  Measurements=None
      settings: SourceProductName=Simscape Electrical
  Controlled Voltage Source1 : powerlib/Electrical Sources/Controlled Voltage Source  Initialize=on  Source_Type=DC  Amplitude=0  Phase=0  Frequency=0  Measurements=None
      settings: SourceProductName=Simscape Electrical
  Diode : powerlib/Power Electronics/Diode  Ron=0.001  Lon=0  Vf=v_ovp  IC=0  UseSnubber=off  Rs=500  Cs=250e-9  Measurements=off
      settings: SourceProductName=Simscape Electrical
  Discrete PID Controller : simulink/Continuous/PID Controller  Controller=PI  Form=Parallel  TimeDomain=Discrete-time  SampleTime=-1  IntegratorMethod=Forward Euler  FilterMethod=Forward Euler  ControllerParametersSource=internal  P=1  I=0.02  D=0  UseFilter=on  N=100  TunerSelectOption=Transfer Function Based (PID Tuner App)  InitialConditionSource=internal  InitialConditionForIntegrator=0  InitialConditionForFilter=0  DifferentiatorICPrevScaledInput=0  ExternalReset=none  TrackingMode=off  Kt=1  LimitOutput=on  UpperSaturationLimit=0.1  LowerSaturationLimit=0  LinearizeAsGain=off  AntiWindupMode=none  Kb=1  POutMin=[]  POutMax=[]  IOutMin=[]  IOutMax=[]  DOutMin=[]  DOutMax=[]  NOutMin=[]  NOutMax=[]  SumOutMin=[]  SumOutMax=[]  SaturationOutMin=[]  SaturationOutMax=[]  PParamMin=[]  PParamMax=[]  IParamMin=[]  IParamMax=[]  DParamMin=[]  DParamMax=[]  NParamMin=[]  NParamMax=[]  KbParamMin=[]  KbParamMax=[]  KtParamMin=[]  KtParamMax=[]  KbOutMin=[]  KbOutMax=[]  KtOutMin=[]  KtOutMax=[]  IntegratorOutMin=[]  IntegratorOutMax=[]  FilterOutMin=[]  FilterOutMax=[]  SumI1OutMin=[]  SumI1OutMax=[]  SumI2OutMin=[]  SumI2OutMax=[]  SumI3OutMin=[]  SumI3OutMax=[]  SumI4OutMin=[]  SumI4OutMax=[]  SumDOutMin=[]  SumDOutMax=[]  DifferentiatorOutMin=[]  DifferentiatorOutMax=[]  FilterDiffOutCoefMin=[]  FilterDiffOutCoefMax=[]  ReciprocalOutMin=[]  ReciprocalOutMax=[]  SumDenOutMin=[]  SumDenOutMax=[]  SumNumOutMin=[]  SumNumOutMax=[]  DivideOutMin=[]  DivideOutMax=[]  IntegratorContinuousStateAttributes=''  IntegratorStateMustResolveToSignalObject=off  IntegratorRTWStateStorageClass=Auto  FilterContinuousStateAttributes=''  FilterStateMustResolveToSignalObject=off  FilterRTWStateStorageClass=Auto  ParallelPVariant=InternalParameters  IdealPVariant=Disabled  IVariant=InternalParameters  DVariant=Disabled  IntegratorVariant=Discrete  SatVariant=Enabled  AWVariant=Passthrough  PCopyVariant=Disabled  TRVariant=Disabled  FdbkBlocksVariant=Forward  IdealPFdbkVariant=Disabled  SatFdbkVariant=Disabled  DerivativeFilterVariant=Disabled  NVariant=Disabled  NCopyVariant=Disabled_SignalSpec  FilterICVariant=Disabled  IntegratorICVariant=InternalICs  ExternalResetVariant=Disabled  TRSumVariant=Passthrough  SumFdbkVariant=Disabled  SumVariant=Sum_PI
  Display : Display
  Gain : Gain  Gain=5
  Memory : Memory  InitialCondition=1  InheritSampleTime=on
  Mosfet : powerlib/Power Electronics/Mosfet  Ron=0.1  Lon=0  Rd=0.01  Vfd=0  IC=0  Rs=1e5  Cs=inf  Measurements=off
      settings: SourceProductName=Simscape Electrical
  Mosfet1 : powerlib/Power Electronics/Mosfet  Ron=0.1  Lon=0  Rd=0.01  Vfd=0  IC=0  Rs=1e5  Cs=inf  Measurements=off
      settings: SourceProductName=Simscape Electrical
  Saturation : Saturate  UpperLimit=inf  LowerLimit=0
  Series RLC Branch : powerlib/Elements/Series RLC Branch  LConnTagsString=__new0  RConnTagsString=__new0  BranchType=R  Resistance=0.001  Inductance=1e-9  SetiL0=off  InitialCurrent=0  Capacitance=1e-6  Setx0=off  InitialVoltage=0  Measurements=None
      settings: SourceProductName=Simscape Electrical
  Sum : Sum  Inputs=|-+
  Switch : Switch  Criteria=u2 > Threshold
  i_cc : powerlib/Measurements/Current Measurement  PhasorSimulation=off  OutputType=Complex  PSBequivalent=0
      settings: SourceProductName=Simscape Electrical
  v_cap_single1 : powerlib/Measurements/Voltage Measurement  PhasorSimulation=off  OutputType=Complex  PSBequivalent=0
      settings: SourceProductName=Simscape Electrical
  V_cc : PMIOPort  Side=Right
  V_ss : PMIOPort  Port=2  Side=Right
  icc : Outport
  vcc : Outport  Port=2
  wires:
  Discrete PID Controller/1 -> Display/1
  Constant/1 -> Sum/2
  Constant1/1 -> Switch/1, Compare To Zero1/1, Saturation/1
  Sum/1 -> Discrete PID Controller/1
  Switch/1 -> Controlled Current Source2/1
  Compare To Zero/1 -> Memory/1
  Memory/1 -> Switch/2
  [vcc] -> Sum/1, Compare To Zero/1
  v_cap_single1/1 -> vcc/1, [vcc]
  i_cc/1 -> icc/1
  Compare To Zero1/1 -> Gain/1
  Gain/1 -> Mosfet1/1, Mosfet/1
  Saturation/1 -> Switch/3
  connections:
  Series RLC Branch/RConn1 -- V_ss/RConn1 -- v_cap_single1/LConn2
  Controlled Current Source2/LConn1 -- Series RLC Branch/LConn1
  v_cap_single1/LConn1 -- Mosfet/RConn1 -- i_cc/RConn1
  i_cc/LConn1 -- V_cc/RConn1
  Mosfet1/RConn1 -- Controlled Current Source2/RConn1
  Mosfet/LConn1 -- Mosfet1/LConn1

== system hybrid_new_eq_circuit_pascal5_single_shot_stack/Protection Circuit 1 ==
  Compare To Constant : simulink/Logic and Bit Operations/Compare To Constant  relop=>  const=v_cut  OutDataTypeStr=uint8
  Compare To Constant1 : simulink/Logic and Bit Operations/Compare To Constant  relop=<  const=v_min  OutDataTypeStr=uint8
  Gain : Gain  Gain=5  OutDataTypeStr=double
  Gain1 : Gain  Gain=5  OutDataTypeStr=double
  Gain2 : Gain  Gain=0  OutDataTypeStr=double
  Mosfet : powerlib/Power Electronics/Mosfet  Ron=0.1  Lon=0  Rd=0.01  Vfd=0  IC=0  Rs=1e5  Cs=inf  Measurements=off
      settings: SourceProductName=Simscape Electrical
  Mosfet1 : powerlib/Power Electronics/Mosfet  Ron=0.1  Lon=0  Rd=0.01  Vfd=0  IC=0  Rs=1e5  Cs=inf  Measurements=off
      settings: SourceProductName=Simscape Electrical
  Rate Limiter : RateLimiter  RisingSlewLimit=d  FallingSlewLimit=-inf  SampleTimeMode=inherited
  Series RLC Branch1 : powerlib/Elements/Series RLC Branch  LConnTagsString=__new0  RConnTagsString=__new0  BranchType=R  Resistance=r  Inductance=1e-3  SetiL0=off  InitialCurrent=0  Capacitance=1e-6  Setx0=off  InitialVoltage=0  Measurements=None
      settings: SourceProductName=Simscape Electrical
  Sum : Sum  Inputs=++|
  i_cc : powerlib/Measurements/Current Measurement  PhasorSimulation=off  OutputType=Complex  PSBequivalent=0
      settings: SourceProductName=Simscape Electrical
  v_cap_single2 : powerlib/Measurements/Voltage Measurement  PhasorSimulation=off  OutputType=Complex  PSBequivalent=0
      settings: SourceProductName=Simscape Electrical
  vcc : PMIOPort  Side=Left
  vss : PMIOPort  Port=2  Side=Left
  vcc1 : PMIOPort  Port=3  Side=Right
  vss1 : PMIOPort  Port=4  Side=Right
  wires:
  Gain1/1 -> Sum/1
  Gain/1 -> Sum/2
  Rate Limiter/1 -> Gain2/1
  Compare To Constant1/1 -> Gain1/1
  Sum/1 -> Rate Limiter/1
  v_cap_single2/1 -> Compare To Constant/1, Compare To Constant1/1
  Compare To Constant/1 -> Gain/1
  Gain2/1 -> Mosfet1/1, Mosfet/1
  connections:
  Series RLC Branch1/RConn1 -- vss1/RConn1 -- v_cap_single2/LConn2 -- vss/RConn1
  Mosfet1/RConn1 -- vcc/RConn1 -- vcc1/RConn1 -- v_cap_single2/LConn1
  Mosfet1/LConn1 -- Mosfet/LConn1
  i_cc/RConn1 -- Mosfet/RConn1
  Series RLC Branch1/LConn1 -- i_cc/LConn1

== system hybrid_new_eq_circuit_pascal5_single_shot_stack/Protection Circuit 2 ==
  Compare To Constant : simulink/Logic and Bit Operations/Compare To Constant  relop=>  const=v_cut  OutDataTypeStr=uint8
  Compare To Constant1 : simulink/Logic and Bit Operations/Compare To Constant  relop=<  const=v_min  OutDataTypeStr=uint8
  Gain : Gain  Gain=5  OutDataTypeStr=double
  Gain1 : Gain  Gain=5  OutDataTypeStr=double
  Gain2 : Gain  Gain=0  OutDataTypeStr=double
  Mosfet : powerlib/Power Electronics/Mosfet  Ron=0.1  Lon=0  Rd=0.01  Vfd=0  IC=0  Rs=1e5  Cs=inf  Measurements=off
      settings: SourceProductName=Simscape Electrical
  Mosfet1 : powerlib/Power Electronics/Mosfet  Ron=0.1  Lon=0  Rd=0.01  Vfd=0  IC=0  Rs=1e5  Cs=inf  Measurements=off
      settings: SourceProductName=Simscape Electrical
  Rate Limiter : RateLimiter  RisingSlewLimit=d  FallingSlewLimit=-inf  SampleTimeMode=inherited
  Series RLC Branch1 : powerlib/Elements/Series RLC Branch  LConnTagsString=__new0  RConnTagsString=__new0  BranchType=R  Resistance=r  Inductance=1e-3  SetiL0=off  InitialCurrent=0  Capacitance=1e-6  Setx0=off  InitialVoltage=0  Measurements=None
      settings: SourceProductName=Simscape Electrical
  Sum : Sum  Inputs=++|
  i_cc : powerlib/Measurements/Current Measurement  PhasorSimulation=off  OutputType=Complex  PSBequivalent=0
      settings: SourceProductName=Simscape Electrical
  v_cap_single2 : powerlib/Measurements/Voltage Measurement  PhasorSimulation=off  OutputType=Complex  PSBequivalent=0
      settings: SourceProductName=Simscape Electrical
  vcc : PMIOPort  Side=Left
  vss : PMIOPort  Port=2  Side=Left
  vcc1 : PMIOPort  Port=3  Side=Right
  vss1 : PMIOPort  Port=4  Side=Right
  wires:
  Gain2/1 -> Mosfet/1, Mosfet1/1
  Compare To Constant/1 -> Gain/1
  v_cap_single2/1 -> Compare To Constant1/1, Compare To Constant/1
  Sum/1 -> Rate Limiter/1
  Compare To Constant1/1 -> Gain1/1
  Rate Limiter/1 -> Gain2/1
  Gain/1 -> Sum/2
  Gain1/1 -> Sum/1
  connections:
  Series RLC Branch1/LConn1 -- i_cc/LConn1
  i_cc/RConn1 -- Mosfet/RConn1
  Mosfet1/LConn1 -- Mosfet/LConn1
  vcc1/RConn1 -- vcc/RConn1 -- Mosfet1/RConn1 -- v_cap_single2/LConn1
  vss1/RConn1 -- v_cap_single2/LConn2 -- vss/RConn1 -- Series RLC Branch1/RConn1

== system hybrid_new_eq_circuit_pascal5_single_shot_stack/Protection Circuit 3 ==
  Compare To Constant : simulink/Logic and Bit Operations/Compare To Constant  relop=>  const=v_cut  OutDataTypeStr=uint8
  Compare To Constant1 : simulink/Logic and Bit Operations/Compare To Constant  relop=<  const=v_min  OutDataTypeStr=uint8
  Gain : Gain  Gain=5  OutDataTypeStr=double
  Gain1 : Gain  Gain=5  OutDataTypeStr=double
  Gain2 : Gain  Gain=0  OutDataTypeStr=double
  Mosfet : powerlib/Power Electronics/Mosfet  Ron=0.1  Lon=0  Rd=0.01  Vfd=0  IC=0  Rs=1e5  Cs=inf  Measurements=off
      settings: SourceProductName=Simscape Electrical
  Mosfet1 : powerlib/Power Electronics/Mosfet  Ron=0.1  Lon=0  Rd=0.01  Vfd=0  IC=0  Rs=1e5  Cs=inf  Measurements=off
      settings: SourceProductName=Simscape Electrical
  Rate Limiter : RateLimiter  RisingSlewLimit=d  FallingSlewLimit=-inf  SampleTimeMode=inherited
  Series RLC Branch1 : powerlib/Elements/Series RLC Branch  LConnTagsString=__new0  RConnTagsString=__new0  BranchType=R  Resistance=r  Inductance=1e-3  SetiL0=off  InitialCurrent=0  Capacitance=1e-6  Setx0=off  InitialVoltage=0  Measurements=None
      settings: SourceProductName=Simscape Electrical
  Sum : Sum  Inputs=++|
  i_cc : powerlib/Measurements/Current Measurement  PhasorSimulation=off  OutputType=Complex  PSBequivalent=0
      settings: SourceProductName=Simscape Electrical
  v_cap_single2 : powerlib/Measurements/Voltage Measurement  PhasorSimulation=off  OutputType=Complex  PSBequivalent=0
      settings: SourceProductName=Simscape Electrical
  vcc : PMIOPort  Side=Left
  vss : PMIOPort  Port=2  Side=Left
  vcc1 : PMIOPort  Port=3  Side=Right
  vss1 : PMIOPort  Port=4  Side=Right
  wires:
  Gain1/1 -> Sum/1
  Gain/1 -> Sum/2
  Rate Limiter/1 -> Gain2/1
  Compare To Constant1/1 -> Gain1/1
  Sum/1 -> Rate Limiter/1
  v_cap_single2/1 -> Compare To Constant/1, Compare To Constant1/1
  Compare To Constant/1 -> Gain/1
  Gain2/1 -> Mosfet1/1, Mosfet/1
  connections:
  Series RLC Branch1/RConn1 -- vss/RConn1 -- v_cap_single2/LConn2 -- vss1/RConn1
  v_cap_single2/LConn1 -- Mosfet1/RConn1 -- vcc/RConn1 -- vcc1/RConn1
  Mosfet1/LConn1 -- Mosfet/LConn1
  i_cc/RConn1 -- Mosfet/RConn1
  Series RLC Branch1/LConn1 -- i_cc/LConn1

== system hybrid_new_eq_circuit_pascal5_single_shot_stack/Supercapacitor 1 ==
  note: 6x 700R
  note: 4x 1k4
  note: 4x 625R
  note: 1x 550R
  note: 1x 4k
  Bus Creator : BusCreator  Inputs=11
  Subsystem : Subsystem  mask{c=c(2), r_esr=r(2), r_leak=r_leak, v_init=v_init2}
      mask prompts: c "Capacitance /F"; r_esr "Series resistance /ohm"; r_leak "Leak resistance /ohm (inf for disabled)"; v_init "Initial capacitor voltage"
  Subsystem1 : Subsystem  mask{c=c(4), r_esr=r(4), r_leak=r_leak, v_init=v_init4}
      mask prompts: c "Capacitance /F"; r_esr "Series resistance /ohm"; r_leak "Leak resistance /ohm (inf for disabled)"; v_init "Initial capacitor voltage"
  Subsystem2 : Subsystem  mask{c=c(3), r_esr=r(3), r_leak=r_leak, v_init=v_init3}
      mask prompts: c "Capacitance /F"; r_esr "Series resistance /ohm"; r_leak "Leak resistance /ohm (inf for disabled)"; v_init "Initial capacitor voltage"
  Subsystem5 : Subsystem  mask{c=c(5), r_esr=r(5), r_leak=r_leak, v_init=v_init5}
      mask prompts: c "Capacitance /F"; r_esr "Series resistance /ohm"; r_leak "Leakage resistance /ohm (inf for disabled)"; v_init "Initial capacitor voltage"
  Subsystem8 : Subsystem  mask{c=c(1), r_esr=r(1), r_leak=r_leak, v_init=v_init1}
      mask prompts: c "Capacitance /F"; r_esr "Series resistance /ohm"; r_leak "Leakage resistance /ohm (inf for disabled)"; v_init "Initial capacitor voltage"
  v_cap_single : powerlib/Measurements/Voltage Measurement  PhasorSimulation=off  OutputType=Complex  PSBequivalent=0
      settings: SourceProductName=Simscape Electrical
  VCC_in : PMIOPort  Side=Left
  VSS_in : PMIOPort  Port=2  Side=Left
  VCC_out : PMIOPort  Port=3  Side=Right
  VSS_out : PMIOPort  Port=4  Side=Right
  v_r_out : Outport
  v_cap_out : Outport  Port=2
  i_leak_out : Outport  Port=3
  p_chg_out : Outport  Port=4
  p_leak_out : Outport  Port=5
  i_out : Outport  Port=6
  c_out : Outport  Port=7
  r_out : Outport  Port=8
  r_leak_out : Outport  Port=9
  bus_out : Outport  Port=10
  wires:
  Subsystem5/5(p_leak_out) -> Bus Creator/5, p_leak_out/1
  Subsystem5/6(i_out) -> Bus Creator/6, i_out/1
  Subsystem5/4(p_chg_out) -> Bus Creator/4, p_chg_out/1
  Subsystem5/7(c_out) -> Bus Creator/7, c_out/1
  Subsystem5/3(i_leak_out) -> Bus Creator/3, i_leak_out/1
  Subsystem5/8(r_out) -> Bus Creator/8, r_out/1
  Subsystem5/2(v_cap_out) -> Bus Creator/2, v_cap_out/1
  Subsystem5/9(r_leak_out) -> Bus Creator/9, r_leak_out/1
  Subsystem5/1(v_r_out) -> Bus Creator/1, v_r_out/1
  Subsystem8/3(i_leak_out) -> Subsystem/3(In3)
  Subsystem8/6(i_out) -> Subsystem/6(In6)
  Subsystem8/9(r_leak_out) -> Subsystem/9(In9)
  Subsystem8/4(p_chg_out) -> Subsystem/4(In4)
  Subsystem8/10(l_out) -> Subsystem/10(In10)
  Subsystem8/8(r_out) -> Subsystem/8(In8)
  Subsystem8/5(p_leak_out) -> Subsystem/5(In5)
  Subsystem8/7(c_out) -> Subsystem/7(In7)
  Subsystem8/1(v_r_out) -> Subsystem/1(In1)
  Subsystem8/2(v_cap_out) -> Subsystem/2(In2)
  Subsystem1/6(Out6) -> Subsystem5/6(i_in)
  Subsystem1/8(Out8) -> Subsystem5/8(r_in)
  Subsystem1/4(Out4) -> Subsystem5/4(p_chg_in)
  Subsystem1/7(Out7) -> Subsystem5/7(c_in)
  Subsystem1/9(Out9) -> Subsystem5/9(r_leak_in)
  Subsystem1/3(Out3) -> Subsystem5/3(i_leak_in)
  Subsystem1/10(Out10) -> Subsystem5/10(l_in)
  Subsystem1/5(Out5) -> Subsystem5/5(p_leak_in)
  Subsystem1/2(Out2) -> Subsystem5/2(v_cap_in)
  Subsystem1/1(Out1) -> Subsystem5/1(v_r_in)
  Subsystem/3(Out3) -> Subsystem2/3(In3)
  Subsystem/10(Out10) -> Subsystem2/10(In10)
  Subsystem/8(Out8) -> Subsystem2/8(In8)
  Subsystem/1(Out1) -> Subsystem2/1(In1)
  Subsystem/2(Out2) -> Subsystem2/2(In2)
  Subsystem/6(Out6) -> Subsystem2/6(In6)
  Subsystem/9(Out9) -> Subsystem2/9(In9)
  Subsystem/7(Out7) -> Subsystem2/7(In7)
  Subsystem/4(Out4) -> Subsystem2/4(In4)
  Subsystem/5(Out5) -> Subsystem2/5(In5)
  Subsystem2/5(Out5) -> Subsystem1/5(In5)
  Subsystem2/8(Out8) -> Subsystem1/8(In8)
  Subsystem2/6(Out6) -> Subsystem1/6(In6)
  Subsystem2/2(Out2) -> Subsystem1/2(In2)
  Subsystem2/10(Out10) -> Subsystem1/10(In10)
  Subsystem2/9(Out9) -> Subsystem1/9(In9)
  Subsystem2/1(Out1) -> Subsystem1/1(In1)
  Subsystem2/3(Out3) -> Subsystem1/3(In3)
  Subsystem2/4(Out4) -> Subsystem1/4(In4)
  Subsystem2/7(Out7) -> Subsystem1/7(In7)
  v_cap_single/1 -> Bus Creator/11
  Subsystem5/10(l_out) -> Bus Creator/10
  Bus Creator/1 -> bus_out/1
  connections:
  Subsystem8/LConn1 -- VCC_in/RConn1
  VSS_in/RConn1 -- Subsystem8/LConn2
  Subsystem8/RConn2 -- Subsystem/LConn2
  Subsystem8/RConn1 -- Subsystem/LConn1
  Subsystem1/RConn2 -- Subsystem5/LConn2
  Subsystem1/RConn1 -- Subsystem5/LConn1
  Subsystem/RConn1 -- Subsystem2/LConn1
  Subsystem/RConn2 -- Subsystem2/LConn2
  Subsystem1/LConn2 -- Subsystem2/RConn2
  Subsystem1/LConn1 -- Subsystem2/RConn1
  VCC_out/RConn1 -- v_cap_single/LConn1 -- Subsystem5/RConn1
  Subsystem5/RConn2 -- v_cap_single/LConn2 -- VSS_out/RConn1
